simulink model "designAirFlowRate"  (R2025b)
settings: Solver=VariableStepAuto  StartTime=0.0  StopTime=0.01  RelTol=1e-3
values from neighbouring files (symbols this model uses):
  n_des = 65000    [computeSpeedSchedule.m]    (also in scheduleIC.m = interp1(sched.P_el_W, sched.n_ref_rpm, P0c, 'linear'))
  PR_des = 4    [computeSpeedSchedule.m]    (also in scheduleIC.m = fzero(f, PR0, optimset('Display','off','TolX',1e-10)))
libraries: nesl_utility x4, fl_lib x1
settings Model: Creator=Alessandro  LastModifiedBy=Alessandro

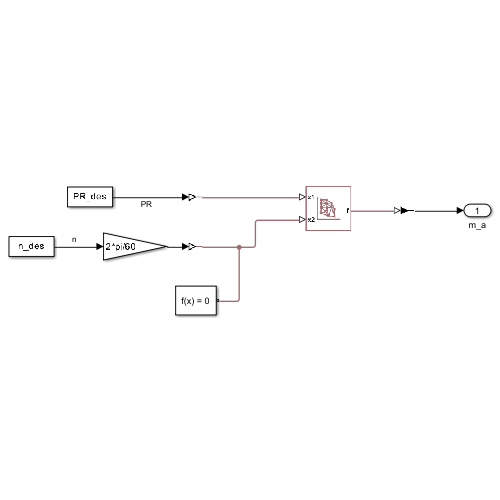
[thumbnail: Simulink's stored preview of the top-level diagram]
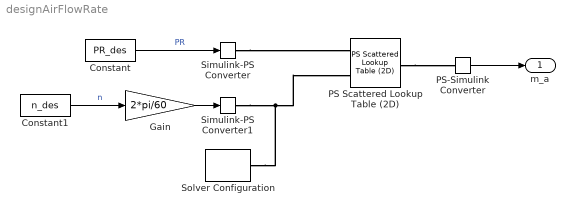
== system designAirFlowRate ==
  Constant : Constant  Value=PR_des
  Constant1 : Constant  Value=n_des
  Gain : Gain  Gain=2*pi/60
  PS Scattered Lookup Table (2D) : fl_lib/Physical Signals/Lookup Tables/PS Scattered Lookup Table (2D)  x1=beta  x2=n rad/s  f=flow kg/s  extrap_method=simscape.enum.extrapolation_slu.linear
      settings: InternalSimscapePortConfiguration="{\"Bottom\":[],\"Left\":[{\"id\":\"I1\",\"label\":\"x1\",\"type\":\"input\"},{\"id\":\"I2\",\"label\":\"x2\",\"type\":\"input\"}],\"Right\":[{\"id\":\"O\",\"label\":\"f\",\"type\":\"output\"}],\"Top\":[]}"
  PS-Simulink Converter : nesl_utility/PS-Simulink Converter  PhysicalDomain=network_engine_domain  SubClassName=ps_output  LeftPortType=input  RightPortType=output  PseudoPeriodic=off  Frequencies=[]  VectorFormat=inherit  Unit=inherit  AffineConversion=off
  Simulink-PS Converter : nesl_utility/Simulink-PS Converter  PhysicalDomain=network_engine_domain  SubClassName=ps_input  LeftPortType=input  RightPortType=output  PseudoPeriodic=off  Frequencies=[]  NoiseDistribution=none  NoiseParameters=[]  Unit=1  AffineConversion=off  FilteringAndDerivatives=provide  SimscapeFilterOrder=1  InputFilterTimeConstant=0.001  UdotUserProvided=0
  Simulink-PS Converter1 : nesl_utility/Simulink-PS Converter  PhysicalDomain=network_engine_domain  SubClassName=ps_input  LeftPortType=input  RightPortType=output  PseudoPeriodic=off  Frequencies=[]  NoiseDistribution=none  NoiseParameters=[]  Unit=rad/s  AffineConversion=off  FilteringAndDerivatives=provide  SimscapeFilterOrder=1  InputFilterTimeConstant=0.001  UdotUserProvided=0
  Solver Configuration : nesl_utility/Solver Configuration  PhysicalDomain=network_engine_domain  SubClassName=solver  LeftPortType=input  RightPortType=generic  Tones=[]  Harmonics=[]  SimulateNoise=off  Profile=off  UseLocalSampling=off  EnableSwitchedLinearOptims=on  FrequencyDomain=off  UseCCode=off  RelTol=0.001  AbsTol=0.001  MinStep=1e-09  ToWorkspace=off  RevertToSquareIcSolve=off  NumHomotopyIterations=100  PhasorMode=off  PhasorModeNumHarmonics=1  ConsistencySolver=NEWTON_XTOL_AFTER_FTOL  IndexReductionMethod=DerivativeReplacement  DoDC=off  ResidualTolerance=1e-09  ConsistencyTolSource=GLOBAL  ConsistencyAbsTol=0.001  ConsistencyRelTol=0.001  ConsistencyTolFactor=0.001  UseLocalSolver=off  LocalSolverChoice=NE_BACKWARD_EULER_ADVANCER  ResolveIndetEquations=on  FunctionEvalNumThread=1  LocalSolverSampleTime=0.001  DoFixedCost=off  MaxNonlinIter=3  MaxModeIter=2  ComputeImpulses=off  ImpulseIterations=2  LinearAlgebra=auto  LinearAlgebraNumThread=0  EquationFormulation=NE_TIME_EF  DelaysMemoryBudget=1024  AutomaticFiltering=on  FilteringTimeConstant=0.001  PartitionStorageMethod=AS_NEEDED  PartitionMemoryBudget=1024  PartitionMethod=ROBUST  MultibodyUseLocalSolver=off  MultibodyLocalSolverChoice=ODE1  MultibodyLocalSolverSampleTime=0.001
  m_a : Outport
  wires:
  Constant1/1 -> Gain/1  "n"
  Constant/1 -> Simulink-PS Converter/1  "PR"
  Gain/1 -> Simulink-PS Converter1/1
  PS-Simulink Converter/1 -> m_a/1
  connections:
  Solver Configuration/RConn1 -- Simulink-PS Converter1/RConn1 -- PS Scattered Lookup Table (2D)/LConn2
  PS Scattered Lookup Table (2D)/RConn1 -- PS-Simulink Converter/LConn1
  Simulink-PS Converter/RConn1 -- PS Scattered Lookup Table (2D)/LConn1
